simulink model "sist_susp_coche_prac3"  (R2025a)
settings: Solver=VariableStepAuto  StartTime=0.0  StopTime=10.0  RelTol=1e-3
InitFcn:
  | m1 = 290;
  | b1 = 1000;
  | m2 = 59;
  | k1 = 16182;
  | f = 0;
  | k2 = 19000;
settings Model: Creator=USER  LastModifiedBy=USER

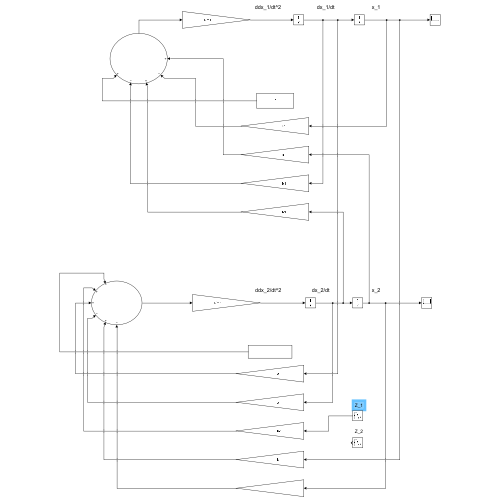
[thumbnail: Simulink's stored preview of the top-level diagram]
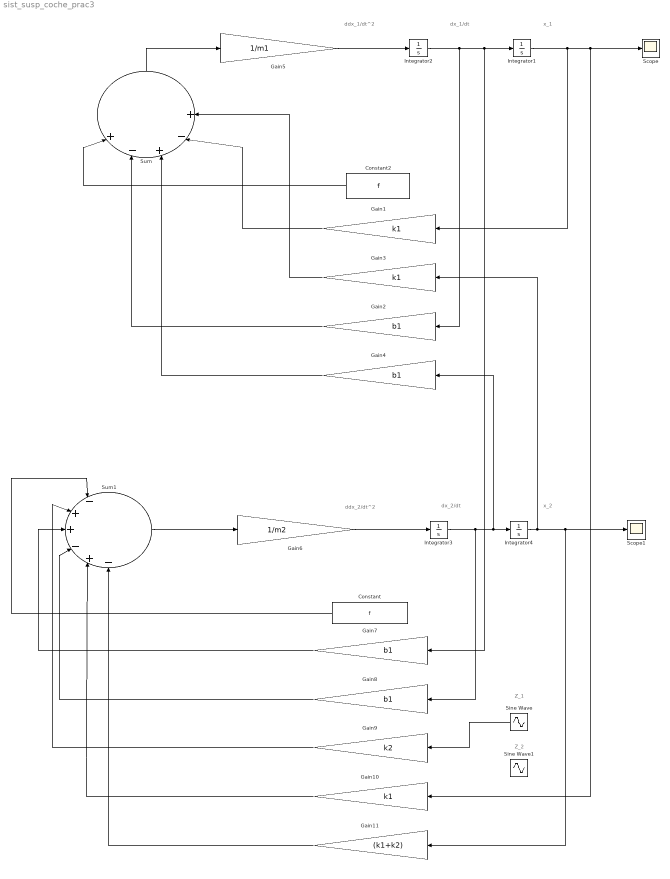
== system sist_susp_coche_prac3 ==
  note: Z_1
  note: ddx_1/dt^2
  note: dx_1/dt
  note: x_1
  note: ddx_2/dt^2
  note: dx_2/dt
  note: x_2
  note: Z_2
  Constant : Constant  Value=f
  Constant2 : Constant  Value=f
  Gain1 : Gain  Gain=k1
  Gain10 : Gain  Gain=k1
  Gain11 : Gain  Gain=(k1+k2)
  Gain{2,4,7..8} (4 alike) : Gain  Gain=b1
  Gain3 : Gain  Gain=k1
  Gain5 : Gain  Gain=1/m1
  Gain6 : Gain  Gain=1/m2
  Gain9 : Gain  Gain=k2
  Integrator{1..4} (4 alike) : Integrator
  Scope : Scope
      settings: ActiveDisplayYMinimum=-0.070240527704496708  ActiveDisplayYMaximum=0.080554855938756692
  Scope1 : Scope
      settings: ActiveDisplayYMinimum=-0.066392429182942844  ActiveDisplayYMaximum=0.070956552851740851
  Sine Wave : Sin  Amplitude=0.05  Frequency=0.5*pi  SampleTime=0
  Sine Wave1 : Sin  Amplitude=0.05  Frequency=20*pi  SampleTime=0
  Sum : Sum  Inputs=|+-+-+
  Sum1 : Sum  Inputs=|-++-+-
  wires:
  Gain5/1 -> Integrator2/1
  Integrator2/1 -> Gain7/1, Integrator1/1, Gain2/1
  Integrator1/1 -> Scope/1, Gain10/1, Gain1/1
  Integrator3/1 -> Gain8/1, Gain4/1, Integrator4/1
  Integrator4/1 -> Scope1/1, Gain11/1, Gain3/1
  Gain6/1 -> Integrator3/1
  Constant2/1 -> Sum/1
  Gain2/1 -> Sum/2
  Gain4/1 -> Sum/3
  Sum/1 -> Gain5/1
  Gain1/1 -> Sum/4
  Gain3/1 -> Sum/5
  Sum1/1 -> Gain6/1
  Constant/1 -> Sum1/1
  Gain9/1 -> Sum1/2
  Gain7/1 -> Sum1/3
  Gain8/1 -> Sum1/4
  Gain10/1 -> Sum1/5
  Gain11/1 -> Sum1/6
  Sine Wave/1 -> Gain9/1
